simulink library "HEV_Electrical_Lib_org"  (Simulink 10.0)
settings: Solver=ode23t  StartTime=0.0  StopTime=10.0  MaxStep=1e-3  RelTol=1e-3
undefined symbols (not defined in the file): DiscIntNeverNeededParam, HEV_Param, magnitude, Ts
libraries: fl_lib x67, powerlib x61, nesl_utility x32, fl_ps_legacy_lib x16, simulink_extras x8, simulink x6, HEV_Battery_Det_Lib x4, electricdrivelib x4, HEV_Battery_Lib x3, powerlib_extras x2, ee_lib x2, $bdroot x1
(part 4 of 4)

== system HEV_Electrical_Lib_org/Mean Value/Synchronous Motor & Drive/Three-phase Inverter/Limit detection ==
  note: Low pass filter
  note: Low pass filter
  note: Limit = 1 saturation mode (voltage mode)
      | Limit = 0 normal mode (current mode)
  Vcc : Inport
  ctrl : Inport  Port=2
  Bus Selector1 : BusSelector  OutputSignals=m.Stator current is_d (A),m.Stator current is_q (A),m.Rotor speed wm (rad/s)  OutputAsBus=on
  Discrete Transfer Fcn1 : DiscreteTransferFcn  Numerator=[1-exp(-Ts*Fcs*2*pi)]  Denominator=[1 -exp(-Ts*Fcs*2*pi)]  SampleTime=Ts
  Discrete Transfer Fcn3 : DiscreteTransferFcn  Numerator=[1-exp(-Ts*Fcs*2*pi)]  Denominator=[1 -exp(-Ts*Fcs*2*pi)]  SampleTime=Ts
  Gain1 : Gain  Gain=0.9  SaturateOnIntegerOverflow=on  OutDataTypeStr=Inherit: Same as input  ParamDataTypeStr=Inherit: Same as input
  "Internal Vcc " : Fcn  Expr=pi/2*sqrt((Resistance*u(1)-Lq*p*u(3)*u(2))^2+(Resistance*u(2)+Ld*p*u(3)*u(1)+Flux*p*u(3))^2)
  Relational Operator : RelationalOperator  Operator=>  OutDataTypeStr=boolean  RndMeth=Nearest
  Relational Operator2 : RelationalOperator  Operator=<  OutDataTypeStr=boolean  RndMeth=Nearest
  S-R Flip-Flop : simulink_extras/Flip Flops/S-R Flip-Flop  initial_condition=0
  Terminator : Terminator
  Limit : Outport
  wires:
  S-R Flip-Flop/2 -> Terminator/1
  Discrete Transfer Fcn3/1 -> Relational Operator/2, Gain1/1
  Gain1/1 -> Relational Operator2/2
  Discrete Transfer Fcn1/1 -> Relational Operator2/1, Relational Operator/1
  "Internal Vcc "/1 -> Discrete Transfer Fcn1/1
  Bus Selector1/1 -> "Internal Vcc "/1
  ctrl/1 -> Bus Selector1/1
  S-R Flip-Flop/1 -> Limit/1
  Relational Operator2/1 -> S-R Flip-Flop/2
  Relational Operator/1 -> S-R Flip-Flop/1
  Vcc/1 -> Discrete Transfer Fcn3/1

== system HEV_Electrical_Lib_org/Mean Value/Synchronous Motor & Drive/Three-phase Inverter/Output Resistance correction ==
  note: Vabc
  ctrl : Inport
  1/R : Gain  Gain=1/(100*Resistance)  SaturateOnIntegerOverflow=on  OutDataTypeStr=Inherit: Same as input  ParamDataTypeStr=Inherit: Same as input
  Bus Selector1 : BusSelector  OutputSignals=m.Stator voltage Vs_d (V),m.Stator voltage Vs_q (V),m.Rotor angle thetam (rad)
  Constant : Constant  Value=0
  Discrete Transfer Fcn1 : DiscreteTransferFcn  Numerator=[1-exp(-Ts/.001)]  Denominator=[1 -exp(-Ts/.001)]  SampleTime=Ts
  Discrete Transfer Fcn2 : DiscreteTransferFcn  Numerator=[1-exp(-Ts/.001)]  Denominator=[1 -exp(-Ts/.001)]  SampleTime=Ts
  Fcn : Fcn  Expr=sin(u)
  Fcn1 : Fcn  Expr=cos(u)
  Mux4 : Mux  Inputs=3
  Mux5 : Mux  Inputs=2
  dq0_to_abc Transformation : powerlib_extras/Measurements/dq0_to_abc Transformation
      settings: SourceProductName=Simscape Electrical  SourceProductBaseCode=PS
  poles : Gain  Gain=p  SaturateOnIntegerOverflow=on  OutDataTypeStr=Inherit: Same as input  ParamDataTypeStr=Inherit: Same as input
  "Iabc_r " : Outport
  wires:
  poles/1 -> Fcn/1, Fcn1/1
  Bus Selector1/3 -> poles/1  "<Rotor angle thetam (rad)>"
  Discrete Transfer Fcn1/1 -> Mux4/1
  Discrete Transfer Fcn2/1 -> Mux4/2
  dq0_to_abc Transformation/1 -> 1/R/1
  Constant/1 -> Mux4/3
  Mux5/1 -> dq0_to_abc Transformation/2
  Fcn1/1 -> Mux5/2
  Fcn/1 -> Mux5/1
  Mux4/1 -> dq0_to_abc Transformation/1
  ctrl/1 -> Bus Selector1/1
  Bus Selector1/1 -> Discrete Transfer Fcn1/1  "<Stator voltage Vs_d (V)>"
  Bus Selector1/2 -> Discrete Transfer Fcn2/1  "<Stator voltage Vs_q (V)>"
  1/R/1 -> "Iabc_r "/1

== system HEV_Electrical_Lib_org/Mean Value/Synchronous Motor & Drive/VECT controller/Current Regulator ==
  Iabc* : Inport
  Iabc : Inport  Port=2
  Demux1 : Demux  Outputs=3
  Demux2 : Demux  Outputs=3
  Mux1 : Mux  Inputs=2
  Relay : Relay  OnSwitchValue=0  OffSwitchValue=0
  Relay1 : Relay  OnSwitchValue=0  OffSwitchValue=0
  Relay2 : Relay  OnSwitchValue=0  OffSwitchValue=0
  Sum : Sum  Inputs=-+  SaturateOnIntegerOverflow=on  InputSameDT=on  OutDataTypeStr=Inherit: Same as first input
  Sum1 : Sum  Inputs=-+  SaturateOnIntegerOverflow=on  InputSameDT=on  OutDataTypeStr=Inherit: Same as first input
  Sum2 : Sum  Inputs=-+  SaturateOnIntegerOverflow=on  InputSameDT=on  OutDataTypeStr=Inherit: Same as first input
  Sum3 : Sum  Inputs=+-
  Sum4 : Sum  Inputs=+-
  Pulses : Outport  InitialOutput=0
  wires:
  Sum4/1 -> Mux1/2
  Sum3/1 -> Mux1/1
  Relay2/1 -> Sum4/2
  Relay1/1 -> Sum4/1, Sum3/2
  Relay/1 -> Sum3/1
  Iabc*/1 -> Demux2/1
  Demux2/1 -> Sum/2
  Demux2/2 -> Sum1/2
  Demux2/3 -> Sum2/2
  Demux1/3 -> Sum2/1
  Sum2/1 -> Relay2/1
  Iabc/1 -> Demux1/1
  Mux1/1 -> Pulses/1
  Demux1/2 -> Sum1/1
  Demux1/1 -> Sum/1
  Sum1/1 -> Relay1/1
  Sum/1 -> Relay/1

== system HEV_Electrical_Lib_org/Mean Value/Synchronous Motor & Drive/VECT controller/DQ-ABC ==
  "Iq* " : Inport
  "Id* " : Inport  Port=2
  Teta : Inport  Port=3
  Fcn : Fcn  Expr=sin(u)
  Fcn1 : Fcn  Expr=cos(u)
  Gain2 : Gain  SaturateOnIntegerOverflow=on  OutDataTypeStr=Inherit: Same as input  ParamDataTypeStr=Inherit: Same as input
  Gain3 : Gain  SaturateOnIntegerOverflow=on  OutDataTypeStr=Inherit: Same as input  ParamDataTypeStr=Inherit: Same as input
  Gain4 : Gain  SaturateOnIntegerOverflow=on  OutDataTypeStr=Inherit: Same as input  ParamDataTypeStr=Inherit: Same as input
  Mux : Mux
  Mux2 : Mux  Inputs=3
  ia : Fcn  Expr=-u[3]*u[2] + u[4]*u[1]
  ib : Fcn  Expr=(-u[1]+1.7320508*u[2])*u[4]*0.5+(u[2]+1.7320508*u[1])*u[3]*0.5
  ic : Sum  Inputs=--  SaturateOnIntegerOverflow=on  InputSameDT=on  OutDataTypeStr=Inherit: Same as first input
  Iabc* : Outport  InitialOutput=0
  wires:
  ib/1 -> ic/1, Gain3/1
  ia/1 -> ic/2, Gain2/1
  Gain2/1 -> Mux2/1
  Gain4/1 -> Mux2/3
  ic/1 -> Gain4/1
  Gain3/1 -> Mux2/2
  "Iq* "/1 -> Mux/4
  "Id* "/1 -> Mux/3
  Teta/1 -> Fcn/1, Fcn1/1
  Mux/1 -> ia/1, ib/1
  Mux2/1 -> Iabc*/1
  Fcn1/1 -> Mux/1
  Fcn/1 -> Mux/2

== system HEV_Electrical_Lib_org/Mean Value/Synchronous Motor & Drive/VECT controller/Zero crossing detector ==
  En : Inport
  Iabc* : Inport  Port=2
  D Latch : simulink_extras/Flip Flops/D Latch
      settings: SourceProductName=Simulink  SourceProductBaseCode=SL
  D Latch1 : simulink_extras/Flip Flops/D Latch
      settings: SourceProductName=Simulink  SourceProductBaseCode=SL
  D Latch2 : simulink_extras/Flip Flops/D Latch
      settings: SourceProductName=Simulink  SourceProductBaseCode=SL
  Data Type Conversion : DataTypeConversion
  Data Type Conversion2 : DataTypeConversion
  Demux : Demux  Outputs=3
  Hit  Crossing : HitCross
  Mux : Mux  Inputs=3
  Terminator : Terminator
  Terminator1 : Terminator
  Terminator2 : Terminator
  Enable : Outport
  wires:
  D Latch2/2 -> Terminator2/1
  D Latch1/2 -> Terminator1/1
  D Latch/2 -> Terminator/1
  Data Type Conversion2/1 -> Enable/1
  Iabc*/1 -> Hit  Crossing/1
  En/1 -> Data Type Conversion/1
  Demux/1 -> D Latch/2
  Mux/1 -> Data Type Conversion2/1
  D Latch2/1 -> Mux/3
  D Latch1/1 -> Mux/2
  D Latch/1 -> Mux/1
  Demux/3 -> D Latch2/2
  Demux/2 -> D Latch1/2
  Hit  Crossing/1 -> Demux/1
  Data Type Conversion/1 -> D Latch2/1, D Latch1/1, D Latch/1

== system HEV_Electrical_Lib_org/System Level/DC-DC Converter/Thermal Model/Subsystem ==
  PS-Simulink Converter1 : nesl_utility/PS-Simulink Converter  PhysicalDomain=network_engine_domain  SubClassName=ps_output  LeftPortType=input  RightPortType=output  PseudoPeriodic=off  Frequencies=[]  Unit=degC  AffineConversion=on
  In : PMIOPort  Side=Left
  Out : PMIOPort  Port=2  Side=Right
  tag scope: DCDC_Power_Loss=global
  wires:
  PS-Simulink Converter1/1 -> [DCDC_Power_Loss]
  connections:
  In/RConn1 -- PS-Simulink Converter1/LConn1 -- Out/RConn1

== system HEV_Electrical_Lib_org/System Level/DC-DC Converter/Thermal Model/Temperature Sensor ==
  Ideal Temperature Sensor : fl_lib/Thermal/Thermal Sensors/Temperature Sensor
  PS-Simulink Converter : nesl_utility/PS-Simulink Converter  PhysicalDomain=network_engine_domain  SubClassName=ps_output  LeftPortType=input  RightPortType=output  PseudoPeriodic=off  Frequencies=[]  Unit=degC  AffineConversion=on
  Thermal Reference : fl_lib/Thermal/Thermal Elements/Thermal Reference
  Conn2 : PMIOPort  Side=Left
  tag scope: DCDC_SYS=global
  wires:
  PS-Simulink Converter/1 -> [DCDC_SYS]  "DCDC_Temp"
  connections:
  PS-Simulink Converter/LConn1 -- Ideal Temperature Sensor/RConn2
  Thermal Reference/LConn1 -- Ideal Temperature Sensor/RConn1
  Conn2/RConn1 -- Ideal Temperature Sensor/LConn1

== system HEV_Electrical_Lib_org/Detailed/DC/DC Converter/PWM/Thermal Model/Subsystem ==
  IBus : Inport
  PToHeat : Gain  Gain=HEV_Param.DCDCConv.EPower2Heat  SaturateOnIntegerOverflow=on  OutDataTypeStr=Inherit: Same as input  ParamDataTypeStr=Inherit: Same as input
  Product : Product  RndMeth=Zero
  RLoss : Gain  Gain=HEV_Param.DCDCConv.Resistance_Losses  SaturateOnIntegerOverflow=on  OutDataTypeStr=Inherit: Same as input  ParamDataTypeStr=Inherit: Same as input
  Heat Flow : Outport
  wires:
  Product/1 -> RLoss/1
  IBus/1 -> Product/1, Product/2
  RLoss/1 -> PToHeat/1
  PToHeat/1 -> Heat Flow/1

== system HEV_Electrical_Lib_org/Mean Value/DC/DC Converter/Boost Converter Average-Values/Thermal Model/Subsystem ==
  IBus : Inport
  PToHeat : Gain  Gain=HEV_Param.DCDCConv.EPower2Heat  SaturateOnIntegerOverflow=on  OutDataTypeStr=Inherit: Same as input  ParamDataTypeStr=Inherit: Same as input
  Product : Product  RndMeth=Zero
  RLoss : Gain  Gain=HEV_Param.DCDCConv.Resistance_Losses  SaturateOnIntegerOverflow=on  OutDataTypeStr=Inherit: Same as input  ParamDataTypeStr=Inherit: Same as input
  Heat Flow : Outport
  wires:
  PToHeat/1 -> Heat Flow/1
  RLoss/1 -> PToHeat/1
  IBus/1 -> Product/2, Product/1
  Product/1 -> RLoss/1

== system HEV_Electrical_Lib_org/Mean Value/Synchronous Generator & Drive/Three-phase Inverter/Id computation/Demux ==
  m : Inport
  Demux1 : Demux  Outputs=5
  Terminator : Terminator
  Vac : Outport
  Ia : Outport  Port=2
  Vbc : Outport  Port=3
  Ib : Outport  Port=4
  wires:
  m/1 -> Demux1/1
  Demux1/5 -> Vbc/1  "Vbc"
  Demux1/4 -> Vac/1  "Vac"
  Demux1/2 -> Ib/1  "Ib"
  Demux1/1 -> Ia/1  "Ia"
  Demux1/3 -> Terminator/1  "Ic"

== system HEV_Electrical_Lib_org/Mean Value/Synchronous Generator & Drive/Three-phase Inverter/Id computation/Demux1 ==
  m : Inport
  Demux1 : Demux  Outputs=5
  Terminator1 : Terminator
  Terminator2 : Terminator
  Ia : Outport
  Ib : Outport  Port=2
  Ic : Outport  Port=3
  wires:
  Demux1/3 -> Ic/1  "Ic"
  Demux1/1 -> Ia/1  "Ia"
  Demux1/2 -> Ib/1  "Ib"
  Demux1/4 -> Terminator1/1  "Vac"
  Demux1/5 -> Terminator2/1  "Vbc"
  m/1 -> Demux1/1

== system HEV_Electrical_Lib_org/Mean Value/Synchronous Motor & Drive/Three-phase Inverter/Id computation/Demux ==
  m : Inport
  Demux1 : Demux  Outputs=5
  Terminator : Terminator
  Vac : Outport
  Ia : Outport  Port=2
  Vbc : Outport  Port=3
  Ib : Outport  Port=4
  wires:
  Demux1/3 -> Terminator/1  "Ic"
  Demux1/1 -> Ia/1  "Ia"
  Demux1/2 -> Ib/1  "Ib"
  Demux1/4 -> Vac/1  "Vac"
  Demux1/5 -> Vbc/1  "Vbc"
  m/1 -> Demux1/1

== system HEV_Electrical_Lib_org/Mean Value/Synchronous Motor & Drive/Three-phase Inverter/Id computation/Demux1 ==
  m : Inport
  Demux1 : Demux  Outputs=5
  Terminator1 : Terminator
  Terminator2 : Terminator
  Ia : Outport
  Ib : Outport  Port=2
  Ic : Outport  Port=3
  wires:
  m/1 -> Demux1/1
  Demux1/5 -> Terminator2/1  "Vbc"
  Demux1/4 -> Terminator1/1  "Vac"
  Demux1/2 -> Ib/1  "Ib"
  Demux1/1 -> Ia/1  "Ia"
  Demux1/3 -> Ic/1  "Ic"

== matlab function Mean Value/Synchronous Motor & Drive/VECT controller/Embedded MATLAB Function1 ==
  data: iqn_opt input double; Ten input double; iqn output double; w input double; Vdc input double; params input double; idn output double
function [iqn,idn] = fcn(iqn_opt,Ten,w,Vdc,params)
% This block supports the Embedded MATLAB subset.
% See the help menu for details.

kFact = 0.9;
Ld = params(1);
Lq = params(2);
lam = params(3);
p = params(4);
ib = params(5);
Vs = Vdc/(pi/2)*kFact;
ten = abs(Ten);
iqn = sign(Ten)*iqn_opt;
if Ten == 0 && w == 0
    idn = 0;
elseif iqn == 0
    idn = -(lam*p*w-Vs*kFact)/(p*Ld*w*ib);
else
    idn = 1-Ten/iqn;
end
if sqrt((-Lq*p*w*iqn*ib)^2+(Ld*p*w*idn*ib+lam*p*w)^2) >= Vs 
    vs = Vs;
    k1 = 2*lam*Ld/(ib*Lq^2);
    k2 = Ld^2/Lq^2;
    k3 = lam^2/(ib^2*Lq^2)+k2;
    
    g2 = -vs^2/(p^2*ib^2*Lq^2*w^2) + k1 + k3;
    g3 = -k1*ten-2*ten*k2;
    g4 = k2*ten^2;
    
    a1 = abs(-768*g4^3+384*g4^2*g2^2-48*g4*g2^4-432*g2*g4*g3^2+81*g3^4+12*g3^2*g2^3)^(1/2);
    a2 = (-288*g2*g4+108*g3^2+8*g2^3+12*a1)^(1/3);
    a3 = (-4*g2+a2+48/a2*g4+4/a2*g2^2)^(1/2);
    iqn = (1/12*6^(1/2)*a3+1/12*abs(-48*g2-6*a2-288/a2*g4-24/a2*g2^2-72/a3*g3*6^(1/2))^(1/2));
    iqn = sign(Ten)*iqn;

    idn = 1-Ten/iqn;
end

== matlab function Detailed/Synchronous Motor & Drive/VECT Controller/Embedded MATLAB Function1 ==
  data: iqn_opt input double; Ten input double; iqn output double; w input double; Vdc input double; params input double; idn output double
function [iqn,idn] = fcn(iqn_opt,Ten,w,Vdc,params)
% This block supports the Embedded MATLAB subset.
% See the help menu for details.

kFact = 0.9;
Ld = params(1);
Lq = params(2);
lam = params(3);
p = params(4);
ib = params(5);
Vs = Vdc/(pi/2)*kFact;
ten = abs(Ten);
iqn = sign(Ten)*iqn_opt;
if Ten == 0 && w == 0
    idn = 0;
elseif iqn == 0
    idn = -(lam*p*w-Vs*kFact)/(p*Ld*w*ib);
else
    idn = 1-Ten/iqn;
end
if sqrt((-Lq*p*w*iqn*ib)^2+(Ld*p*w*idn*ib+lam*p*w)^2) >= Vs 
    vs = Vs;
    k1 = 2*lam*Ld/(ib*Lq^2);
    k2 = Ld^2/Lq^2;
    k3 = lam^2/(ib^2*Lq^2)+k2;
    
    g2 = -vs^2/(p^2*ib^2*Lq^2*w^2) + k1 + k3;
    g3 = -k1*ten-2*ten*k2;
    g4 = k2*ten^2;
    
    a1 = abs(-768*g4^3+384*g4^2*g2^2-48*g4*g2^4-432*g2*g4*g3^2+81*g3^4+12*g3^2*g2^3)^(1/2);
    a2 = (-288*g2*g4+108*g3^2+8*g2^3+12*a1)^(1/3);
    a3 = (-4*g2+a2+48/a2*g4+4/a2*g2^2)^(1/2);
    iqn = (1/12*6^(1/2)*a3+1/12*abs(-48*g2-6*a2-288/a2*g4-24/a2*g2^2-72/a3*g3*6^(1/2))^(1/2));
    iqn = sign(Ten)*iqn;

    idn = 1-Ten/iqn;
end
